simulink model "ServerExp_Model"  (R2023a)
settings: Solver=VariableStepAuto  StartTime=0.0  StopTime=10.0  RelTol=1e-3
libraries: NSA_DEVS_SINKS_ATOMIC x5, TimeSharedLib x4, NSA_DEVS_LOGISTICS_ATOMIC x2, NSA_DEVS_SOURCES_ATOMIC x1
settings Model: Creator=david  LastModifiedBy=peter

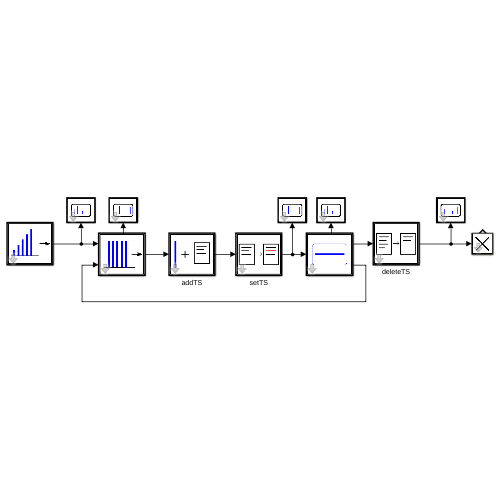
[thumbnail: Simulink's stored preview of the top-level diagram]
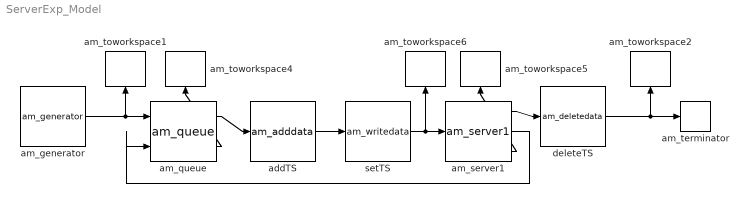
== system ServerExp_Model ==
  addTS : TimeSharedLib/am_adddata  fields="[\"serviceTime\"]"  values="[\"1\"]"  numeric=[true]  infield="\"id\""  tau=[0,0.25]  debug=0
  am_generator : NSA_DEVS_SOURCES_ATOMIC/am_generator  tG=1  n0=1  nG=10  tau=[0,1]  debug=0
      settings: SourceProductName=NSA_DEVS
  am_queue : NSA_DEVS_LOGISTICS_ATOMIC/am_queue  tD=[0,2]  tau=[0,1]  debug=0
      settings: SourceProductName=NSA_DEVS
  am_server1 : TimeSharedLib/am_server1  tS=1.0  tsField="\"serviceTime\""  tau=[0,0.25]  debug=0
  am_terminator : NSA_DEVS_LOGISTICS_ATOMIC/am_terminator  tau=[0,1]  debug=0
      settings: SourceProductName=NSA_DEVS
  am_toworkspace1 : NSA_DEVS_SINKS_ATOMIC/am_toworkspace  varname="\"genOut\""  t0=0  format="\"vector\""  tau=[0,3]  debug=0
      settings: SourceProductName=NSA_DEVS
  am_toworkspace2 : NSA_DEVS_SINKS_ATOMIC/am_toworkspace  varname="\"srvOut\""  t0=0  format="\"vector\""  tau=[0,3]  debug=0
      settings: SourceProductName=NSA_DEVS
  am_toworkspace4 : NSA_DEVS_SINKS_ATOMIC/am_toworkspace  varname="\"nqOut\""  t0=0  format="\"vector\""  tau=[0,3]  debug=0
      settings: SourceProductName=NSA_DEVS
  am_toworkspace5 : NSA_DEVS_SINKS_ATOMIC/am_toworkspace  varname="\"nsOut\""  t0=0  format="\"vector\""  tau=[0,5]  debug=0
      settings: SourceProductName=NSA_DEVS
  am_toworkspace6 : NSA_DEVS_SINKS_ATOMIC/am_toworkspace  varname="\"srvIn\""  t0=0  format="\"vector\""  tau=[0,3]  debug=0
      settings: SourceProductName=NSA_DEVS
  deleteTS : TimeSharedLib/am_deletedata  fields="\"serviceTime\""  tau=[0,0.25]  debug=0
  setTS : TimeSharedLib/am_writedata  inFields=[]  outField="\"serviceTime\""  changeFunc="\"out = -0.9*log(rand());\""  tau=[0,0.25]  debug=0
  wires:
  am_generator/1 -> am_queue/1, am_toworkspace1/1
  am_queue/2 -> am_toworkspace4/1
  setTS/1 -> am_toworkspace6/1, am_server1/1
  am_server1/1 -> deleteTS/1
  addTS/1 -> setTS/1
  am_server1/3 -> am_toworkspace5/1
  am_queue/1 -> addTS/1
  am_server1/2 -> am_queue/2
  deleteTS/1 -> am_toworkspace2/1, am_terminator/1
